simulink model "two_joint_arm"  (R2021a)
settings: Solver=VariableStepAuto  StartTime=0.0  StopTime=inf  RelTol=1e-3
libraries: simulink x2, vrlib x1
settings Model: Creator=kbhar  LastModifiedBy=kbhar

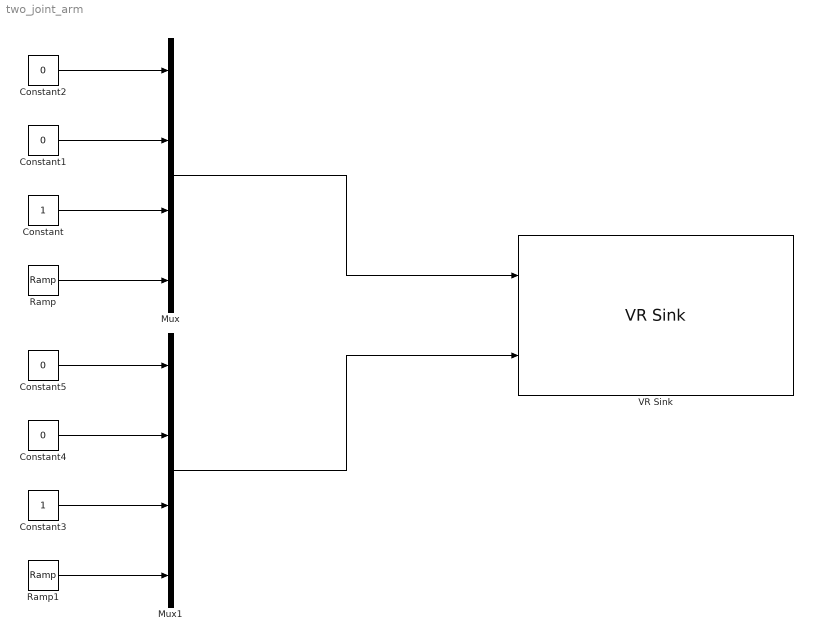
== system two_joint_arm ==
  Constant : Constant
  Constant{1..2,4..5} (4 alike) : Constant  Value=0
  Constant3 : Constant
  Mux : Mux
  Mux1 : Mux
  Ramp : simulink/Sources/Ramp  slope=0.001  start=0  InitialOutput=0
  Ramp1 : simulink/Sources/Ramp  slope=0.01  start=0  InitialOutput=0
  VR Sink : vrlib/VR Sink  InstantiateOnLoad=on  SampleTime=0.1  ViewEnable=on  RemoteChange=off  RemoteView=off  FieldsWritten=shoulder_joint.rotation.4.1.1.double#elbow_joint.rotation.4.1.1.double  WorldFileName=C:\Bharat\College\Projects\Arm Control\Files\test_two_joint_arm.wrl  AutoView=off  VideoDimensions=[]  AllowVariableSize=off
  wires:
  Mux/1 -> VR Sink/1
  Mux1/1 -> VR Sink/2
  Constant/1 -> Mux/3
  Constant2/1 -> Mux/1
  Constant1/1 -> Mux/2
  Constant4/1 -> Mux1/2
  Constant5/1 -> Mux1/1
  Constant3/1 -> Mux1/3
  Ramp/1 -> Mux/4
  Ramp1/1 -> Mux1/4
